simulink model "Reaction_wheel_test"  (R2022b)
settings: Solver=VariableStepAuto  StartTime=0.0  StopTime=10.0  RelTol=1e-3
undefined symbols (not defined in the file): B, Iw, Ke, Kt, La, Ra
settings Model: Creator=Personal  LastModifiedBy=Personal

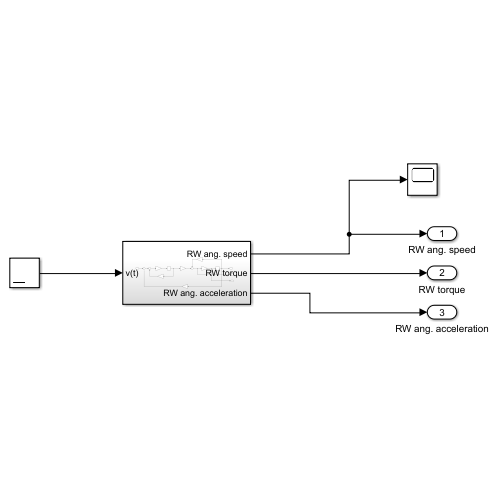
[thumbnail: Simulink's stored preview of the top-level diagram]
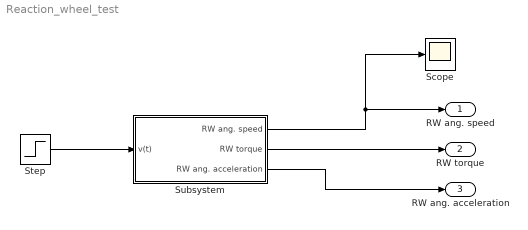
== system Reaction_wheel_test ==
  Scope : Scope
  Step : Step  Time=2  After=12  SampleTime=0
  Subsystem : Subsystem
  RW ang. speed : Outport  VectorParamsAs1DForOutWhenUnconnected=off
  RW torque : Outport  Port=2  VectorParamsAs1DForOutWhenUnconnected=off
  RW ang. acceleration : Outport  Port=3  VectorParamsAs1DForOutWhenUnconnected=off
  wires:
  Step/1 -> Subsystem/1(v(t))
  Subsystem/1(RW ang. speed) -> Scope/1, RW ang. speed/1
  Subsystem/2(RW torque) -> RW torque/1
  Subsystem/3(RW ang. acceleration) -> RW ang. acceleration/1

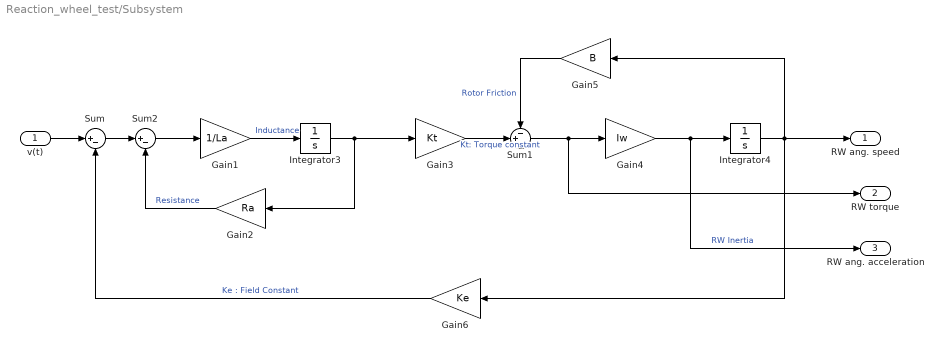
== system Reaction_wheel_test/Subsystem ==
  v(t) : Inport
  Gain1 : Gain  Gain=1/La
  Gain2 : Gain  Gain=Ra
  Gain3 : Gain  Gain=Kt
  Gain4 : Gain  Gain=Iw
  Gain5 : Gain  Gain=B
  Gain6 : Gain  Gain=Ke
  Integrator3 : Integrator
  Integrator4 : Integrator
  Sum : Sum  Inputs=|+-
  Sum1 : Sum  Inputs=-+|
  Sum2 : Sum  Inputs=|+-
  RW ang. speed : Outport  VectorParamsAs1DForOutWhenUnconnected=off
  RW torque : Outport  Port=2  VectorParamsAs1DForOutWhenUnconnected=off
  RW ang. acceleration : Outport  Port=3  VectorParamsAs1DForOutWhenUnconnected=off
  wires:
  Sum/1 -> Sum2/1
  Gain3/1 -> Sum1/2  "Kt: Torque constant"
  Gain1/1 -> Integrator3/1  "Inductance"
  Gain4/1 -> RW ang. acceleration/1, Integrator4/1  "RW Inertia"
  Integrator4/1 -> RW ang. speed/1, Gain6/1, Gain5/1
  Sum1/1 -> RW torque/1, Gain4/1
  Sum2/1 -> Gain1/1
  v(t)/1 -> Sum/1
  Gain5/1 -> Sum1/1  "Rotor Friction"
  Gain6/1 -> Sum/2  "Ke : Field Constant"
  Integrator3/1 -> Gain3/1, Gain2/1
  Gain2/1 -> Sum2/2  "Resistance"
